simulink model "dif_robot"  (R2014b)
settings: Solver=ode45  StartTime=0.0  StopTime=10.0  RelTol=1e-3
settings Model: Creator=mcorberan  LastModifiedBy=samati

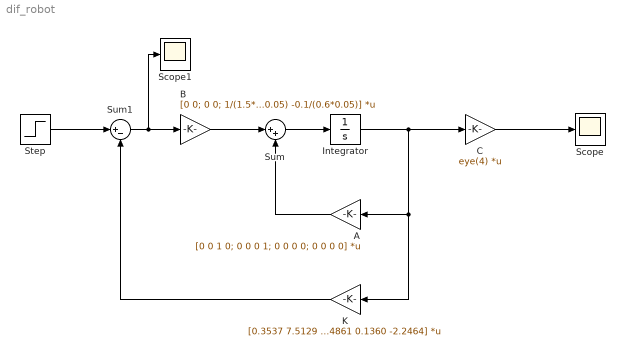
== system dif_robot ==
  A : Gain  Gain=[0 0 1 0; 0 0 0 1; 0 0 0 0; 0 0 0 0]  Multiplication=Matrix(K*u)
  B : Gain  Gain=[0 0; 0 0; 1/(1.5*0.05) 1/(1.5*0.05); 0.1/(0.6*0.05) -0.1/(0.6*0.05)]  Multiplication=Matrix(K*u)
  C : Gain  Gain=eye(4)  Multiplication=Matrix(K*u)
  Integrator : Integrator  InitialCondition=[1; 0; 0; 0]
  K : Gain  Gain=[0.3537 7.5129 0.1641 2.2534; 0.2465 -7.4861 0.1360 -2.2464]  Multiplication=Matrix(K*u)
  Scope : Scope
      settings: ShowLegends=on  YMin=0  YMax=1
  Scope1 : Scope
      settings: ShowLegends=on
  Step : Step  Before=[0; 0]  After=[0; 0]  SampleTime=0  VectorParams1D=off
  Sum : Sum  Inputs=|++
  Sum1 : Sum  Inputs=|+-
  wires:
  A/1 -> Sum/2
  B/1 -> Sum/1
  Sum/1 -> Integrator/1
  Integrator/1 -> K/1, A/1, C/1
  C/1 -> Scope/1
  K/1 -> Sum1/2
  Sum1/1 -> Scope1/1, B/1
  Step/1 -> Sum1/1
